simulink model "BLDC_Openloop"  (R2013a)
settings: Solver=ode45  StartTime=0.0  StopTime=0.5  RelTol=1e-3
undefined symbols (not defined in the file or in its folder): DiscIntNeverNeededParam
libraries: simulink x45, powerlib_meascontrol x11, powerlib x9
settings Model: Creator=Sony  LastModifiedBy=Sony

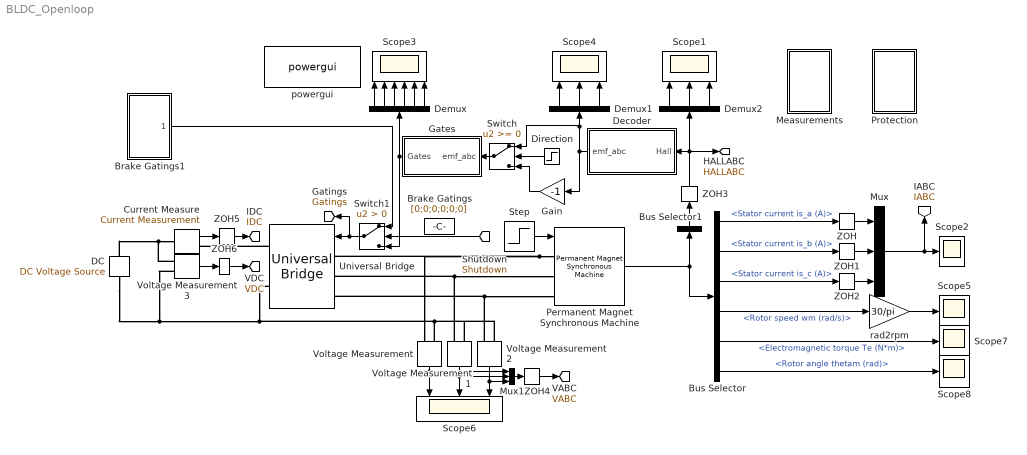
== system BLDC_Openloop ==
  Brake Gatings : Constant  Value=[0;0;0;0;0;0]
  Brake Gatings1 : Subsystem
  Bus Selector : BusSelector  OutputSignals=Stator current is_a (A),Stator current is_b (A),Stator current is_c (A),Rotor speed wm (rad/s),Electromagnetic torque Te (N*m),Rotor angle thetam (rad)
  Bus Selector1 : BusSelector  OutputSignals=Hall effect signal h_a,Hall effect signal h_b,Hall effect signal h_c  OutputAsBus=on
  Current Measure : powerlib/Measurements/Current Measurement  PhasorSimulation=off  OutputType=Complex  PSBequivalent=0
  DC : powerlib/Electrical Sources/DC Voltage Source  Amplitude=48  Measurements=None
  Decoder : Subsystem
  Demux : Demux  Outputs=6
  Demux1 : Demux  Outputs=3
  Demux2 : Demux  Outputs=3
  Direction : Step  Time=.25  Before=1  After=-1  SampleTime=0
  Gain : Gain  Gain=-1
  Gates : Subsystem
  Measurements : Subsystem  mask{Ts=1e-4, Rs=0.01, Ls=1e-4, P=4}
      mask prompts: Ts "Sample Time"; Rs "Stator Resistance"; Ls "Stator Inductance"; P "Pole Pairs"
  Mux : Mux  Inputs=3
  Mux1 : Mux  Inputs=3
  Permanent Magnet Synchronous Machine : powerlib/Machines/Permanent Magnet Synchronous Machine  NbPhases=3  FluxDistribution=Trapezoidal  RotorType=Round  MechanicalLoad=Torque Tm  PresetModel=No  ShowDetailedParameters=on  Resistance=0.01  Inductance=1e-4  dqInductances=[8.5e-3,8.5e-3]  La=0.000835  MachineConstant=Torque Constant (N.m / A_peak)  Flux=0.0125  VoltageCst=10.472  TorqueCst=0.1  Flat=120  Mechanical=[ 1e-3, 1e-7 4]  PolePairs=4  InitialConditions=[(2000)*(pi/30),0, 0,0]  InitialConditions5ph=[0 0 0 0 0 0]  TsPowergui=0  TsBlock=-1  RefAngle=Aligned with phase A axis (original Park)
  Protection : Subsystem  mask{Iphasepeakmax=100, Iphasepeakmin=-100, VDCmax=55, VDCmin=40, IDCmax=125, IDCmin=-125, Accelerationmax=1e7, Accelerationmin=-1e7, VDCrated=48, Temperaturemax=100, Stalltimemax=1, Speedmax=7000, Risetimemax=1e-3}
      mask prompts: Iphasepeakmax "Maximum Phase Peak Current (A)"; Iphasepeakmin "Minimum Phase Peak Current (A)"; VDCmax "Maximum input DC Voltage (V)"; VDCmin "Minimum input DC Voltage (V)"; IDCmax "Maximum input DC Current (A)"; IDCmin "Minimum input DC Current (A)"; Accelerationmax "Maximum Acceleration (rpm/s)"; Accelerationmin "Maximum Deceleration (rpm/s)"; VDCrated "Rated DC input voltage (V)"; Temperaturemax "Maximum Temperature (C)"; Stalltimemax "Maximum Allowed Stall Time (s)"; Speedmax "Maximum Speed (rpm)"; Risetimemax "Maximum MOSFET switch on time (s)"
  Scope1 : Scope  NumInputPorts=3
      settings: YMin=-0.5~-0.5~-0.5  YMax=1.5~1.5~1.5  SaveName=ScopeData3
  Scope{2,5,7..8} (4 alike) : Scope
      Scope2 settings: YMin=-200  YMax=200
      Scope5 settings: YMin=0  YMax=5000  SaveName=ScopeData5
      Scope7 settings: YMin=0  YMax=70  SaveName=ScopeData9
      Scope8 settings: YMin=0  YMax=20  SaveName=ScopeData13
  Scope3 : Scope  NumInputPorts=6
      settings: YMin=-0.5~-0.5~-0.5~-0.5~-0.5~-0.5  YMax=1.5~1.5~1.5~1.5~1.5~1.5
  Scope4 : Scope  NumInputPorts=3
      settings: YMin=-1.5~-1.5~-1.5  YMax=1.5~1.5~1.5  SaveName=ScopeData4
  Scope6 : Scope  NumInputPorts=3
      settings: YMin=-10~-10~-10  YMax=50~50~50  SaveName=ScopeData2
  Step : Step  Time=0.1  After=0  SampleTime=0
  Switch : Switch
  Switch1 : Switch  Criteria=u2 > Threshold
  Universal Bridge : powerlib/Power Electronics/Universal Bridge  Arms=3  SnubberResistance=5000  SnubberCapacitance=1e-6  Device=MOSFET / Diodes  Ron=1e-3  Lon=0  ForwardVoltages="[  0  0  ]"  ForwardVoltage=0  GTOparameters=[ 10e-6 , 20e-6 ]  IGBTparameters=[ 1e-6 , 2e-6 ]  Measurements=None  Measurements_2=None  converterType=Rectifier
  Voltage Measurement{,1..3} (4 alike) : powerlib/Measurements/Voltage Measurement  PhasorSimulation=off  OutputType=Complex  PSBequivalent=0
  ZOH{,1..6} (7 alike) : ZeroOrderHold  SampleTime=1e-4
  powergui : powerlib/powergui  Priority=2  SimulationMode=Discrete  SolverType=Backward Euler  SampleTime=1e-6  frequency=60  SPID=off  DisableSnubberDevices=off  DisableRonSwitches=off  DisableVfSwitches=off  SwTol=0  Interpol=off  DisplayEquations=off  frequencyindice=0  Pbase=100e6  ErrMax=1e-4  Iterations=50  UnitsV=kV  UnitsW=MW  FunctionMessages=off  echomessages=off  HookPort=off  EnableUseOfTLC=off  x0status=blocks  RestoreLinks=warning  ResistiveCurrentMeasurement=off  Frange=[0:2:500]  Ylog=off  Xlog=on  ShowGrid=off  save=off  variable=ZData  ZoomFFT=on  StartTime=0.0  cycles=1  DisplayStyle=1  fundamental=60  FreqAxis=off  MaxFrequency=1000  frequencyindicesteady=1  RmsSteady=1  display=off  Ts=0  methode=off
  rad2rpm : Gain  Gain=30/pi
  tag scope: Gatings=global, HALLABC=global, IABC=global, IDC=global, VABC=global, VDC=global
  wires:
  Step/1 -> Permanent Magnet Synchronous Machine/1
  Gates/1(Gates) -> Switch1/3, Demux/1
  Decoder/1(emf_abc) -> Switch/1, Demux1/1, Gain/1
  rad2rpm/1 -> Scope5/1
  Voltage Measurement/1 -> Mux1/1, Scope6/1
  Bus Selector/1 -> ZOH/1  "<Stator current is_a (A)>"
  Permanent Magnet Synchronous Machine/1 -> Bus Selector/1, Bus Selector1/1
  Bus Selector/2 -> ZOH1/1  "<Stator current is_b (A)>"
  Bus Selector/4 -> rad2rpm/1  "<Rotor speed wm (rad/s)>"
  Demux/3 -> Scope3/3
  Demux/2 -> Scope3/2
  Demux/1 -> Scope3/1
  Demux/4 -> Scope3/4
  Demux/5 -> Scope3/5
  Demux/6 -> Scope3/6
  Demux1/3 -> Scope4/3
  Demux1/2 -> Scope4/2
  Demux1/1 -> Scope4/1
  Demux2/3 -> Scope1/3
  Demux2/2 -> Scope1/2
  Demux2/1 -> Scope1/1
  Bus Selector/3 -> ZOH2/1  "<Stator current is_c (A)>"
  Gain/1 -> Switch/3
  Switch/1 -> Gates/1("emf_abc ")
  Direction/1 -> Switch/2
  Mux/1 -> Scope2/1, [IABC]
  Voltage Measurement1/1 -> Scope6/2, Mux1/2
  Voltage Measurement2/1 -> Scope6/3, Mux1/3
  ZOH/1 -> Mux/1
  ZOH1/1 -> Mux/2
  ZOH2/1 -> Mux/3
  Mux1/1 -> ZOH4/1
  Bus Selector1/1 -> ZOH3/1
  ZOH3/1 -> Demux2/1, [HALLABC], Decoder/1("Hall ")
  Current Measure/1 -> ZOH5/1
  ZOH4/1 -> [VABC]
  Voltage Measurement3/1 -> ZOH6/1
  Bus Selector/5 -> Scope7/1  "<Electromagnetic torque Te (N*m)>"
  ZOH5/1 -> [IDC]
  ZOH6/1 -> [VDC]
  Bus Selector/6 -> Scope8/1  "<Rotor angle thetam (rad)>"
  [Shutdown] -> Switch1/2
  Switch1/1 -> [Gatings], Universal Bridge/1
  Brake Gatings1/1(Gatings) -> Switch1/1
  connections:
  Permanent Magnet Synchronous Machine/LConn1 -- Universal Bridge/LConn1 -- Voltage Measurement/LConn1
  Voltage Measurement1/LConn1 -- Universal Bridge/LConn2 -- Permanent Magnet Synchronous Machine/LConn2
  Voltage Measurement2/LConn1 -- Universal Bridge/LConn3 -- Permanent Magnet Synchronous Machine/LConn3
  DC/RConn1 -- Voltage Measurement3/LConn1 -- Current Measure/LConn1
  DC/LConn1 -- Voltage Measurement3/LConn2 -- Universal Bridge/RConn2 -- Voltage Measurement/LConn2 -- Voltage Measurement1/LConn2 -- Voltage Measurement2/LConn2
  Universal Bridge/RConn1 -- Current Measure/RConn1

== system BLDC_Openloop/Brake Gatings1 ==
  Brake Gatings : Constant  Value=[1;1;1]
  Compare To Zero : simulink/Logic and Bit Operations/Compare To Zero  relop=>=  OutDataTypeStr=boolean
  Constant : Constant  Value=0
  Gates : Subsystem
  Sum2 : Sum  Inputs=|+-
  TRI : powerlib_meascontrol/Pulse & Signal Generators/Triangle Generator  Freq=1e4  Phase=0  Ts=0
  Gatings : Outport
  wires:
  Compare To Zero/1 -> Gates/2(PWM)
  Gates/1(Gates) -> Gatings/1
  Sum2/1 -> Compare To Zero/1
  TRI/1 -> Sum2/2
  Brake Gatings/1 -> Gates/1("emf_abc ")
  Constant/1 -> Sum2/1

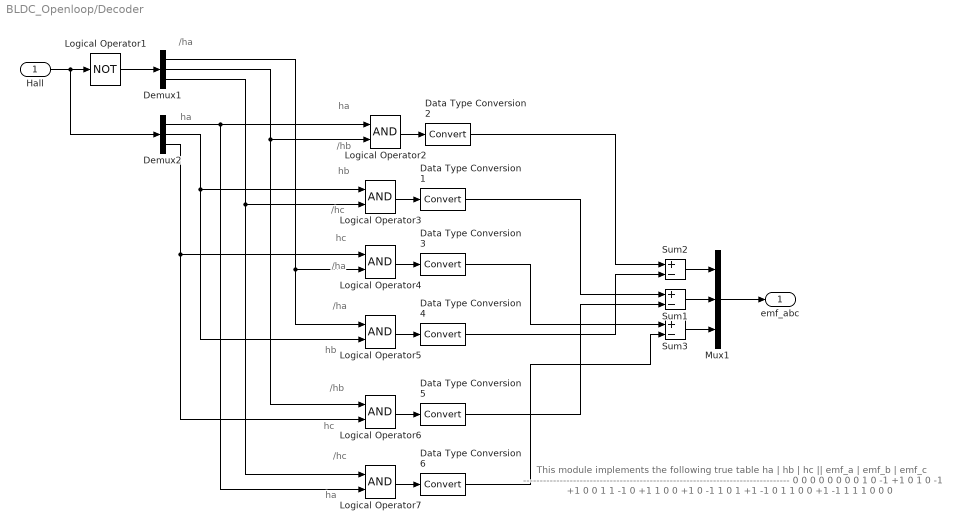
== system BLDC_Openloop/Decoder ==
  note: /ha
  note: ha
  note: ha
  note: /hb
  note: hb
  note: /hc
  note: hc
  note: /ha
  note: /ha
  note: hb
  note: /hb
  note: hc
  note: /hc
  note: ha
  note: This module implements the following true table
      |
      |    ha   |   hb   |   hc   ||   emf_a   |   emf_b   |   emf_c
      |     --------------------------------------------------------------------------------
      | 0          0         0          0               0               0
      | 0          0         1          0               -1              +1
      | 0          1         0          -1              +1                0
      | 0          1         1          -1               0               +1
      | 1          0         0         +1               0               -1
      | 1          0         1         +1              -1                0
      | 1          1         0          0              +1               -1
      | 1          1         1          0               0                0
  "Hall " : Inport
  Data Type Conversion{1..6} (6 alike) : DataTypeConversion
  Demux1 : Demux  Outputs=3
  Demux2 : Demux  Outputs=3
  Logical Operator1 : Logic  Operator=NOT  AllPortsSameDT=off  OutDataTypeStr=boolean
  Logical Operator{2..7} (6 alike) : Logic  AllPortsSameDT=off  OutDataTypeStr=boolean
  Mux1 : Mux  Inputs=3
  Sum1 : Sum  Inputs=+-  OutDataTypeStr=double
  Sum2 : Sum  Inputs=+-  OutDataTypeStr=double
  Sum3 : Sum  Inputs=+-  OutDataTypeStr=double
  emf_abc : Outport
  wires:
  "Hall "/1 -> Logical Operator1/1, Demux2/1
  Logical Operator1/1 -> Demux1/1
  Demux2/3 -> Logical Operator4/1, Logical Operator6/2
  Demux2/2 -> Logical Operator3/1, Logical Operator5/2
  Demux2/1 -> Logical Operator2/1, Logical Operator7/2
  Demux1/3 -> Logical Operator3/2, Logical Operator7/1
  Demux1/2 -> Logical Operator2/2, Logical Operator6/1
  Demux1/1 -> Logical Operator4/2, Logical Operator5/1
  Logical Operator2/1 -> Data Type Conversion2/1
  Sum2/1 -> Mux1/1
  Sum1/1 -> Mux1/2
  Sum3/1 -> Mux1/3
  Mux1/1 -> emf_abc/1
  Logical Operator3/1 -> Data Type Conversion1/1
  Logical Operator4/1 -> Data Type Conversion3/1
  Logical Operator5/1 -> Data Type Conversion4/1
  Logical Operator6/1 -> Data Type Conversion5/1
  Logical Operator7/1 -> Data Type Conversion6/1
  Data Type Conversion2/1 -> Sum2/1
  Data Type Conversion4/1 -> Sum2/2
  Data Type Conversion1/1 -> Sum1/1
  Data Type Conversion5/1 -> Sum1/2
  Data Type Conversion3/1 -> Sum3/1
  Data Type Conversion6/1 -> Sum3/2

== system BLDC_Openloop/Gates ==
  note: This module implements the following true table
      |
      |    emf_a   |   emf_b   |   emf_c   ||   Q1   |   Q2   |   Q3   |   Q4   |   Q5   |   Q6
      |     ------------------------------------------------------------------------------------------------------------------
      |       0              0                0            0          0          0           0        0        0
      |       0               -1              +1          0          0          0           1        1        0
      |     -1              +1                0          0          1          1           0        0        0
      |     -1               0               +1          0          1         0           0        1        0
      |    +1               0                -1          1          0          0           0        0        1
      |    +1              -1                0           1          0          0           1        0        0
      |      0              +1               -1           0          0          1           0        0        1
      |     0              0                0             0          0          0           0        0        0
  "emf_abc " : Inport
  Compare To Zero : simulink/Logic and Bit Operations/Compare To Zero  relop=>  OutDataTypeStr=boolean  ZeroCross=off
  Compare To Zero1 : simulink/Logic and Bit Operations/Compare To Zero  relop=<  OutDataTypeStr=boolean  ZeroCross=off
  Compare To Zero2 : simulink/Logic and Bit Operations/Compare To Zero  relop=>  OutDataTypeStr=boolean  ZeroCross=off
  Compare To Zero3 : simulink/Logic and Bit Operations/Compare To Zero  relop=<  OutDataTypeStr=boolean  ZeroCross=off
  Compare To Zero4 : simulink/Logic and Bit Operations/Compare To Zero  relop=>  OutDataTypeStr=boolean  ZeroCross=off
  Compare To Zero5 : simulink/Logic and Bit Operations/Compare To Zero  relop=<  OutDataTypeStr=boolean  ZeroCross=off
  Demux2 : Demux  Outputs=3
  Mux3 : Mux  Inputs=6
  Gates : Outport
  wires:
  "emf_abc "/1 -> Demux2/1
  Mux3/1 -> Gates/1
  Demux2/1 -> Compare To Zero/1, Compare To Zero1/1
  Demux2/2 -> Compare To Zero2/1, Compare To Zero3/1
  Demux2/3 -> Compare To Zero4/1, Compare To Zero5/1
  Compare To Zero/1 -> Mux3/1
  Compare To Zero1/1 -> Mux3/2
  Compare To Zero2/1 -> Mux3/3
  Compare To Zero3/1 -> Mux3/4
  Compare To Zero4/1 -> Mux3/5
  Compare To Zero5/1 -> Mux3/6

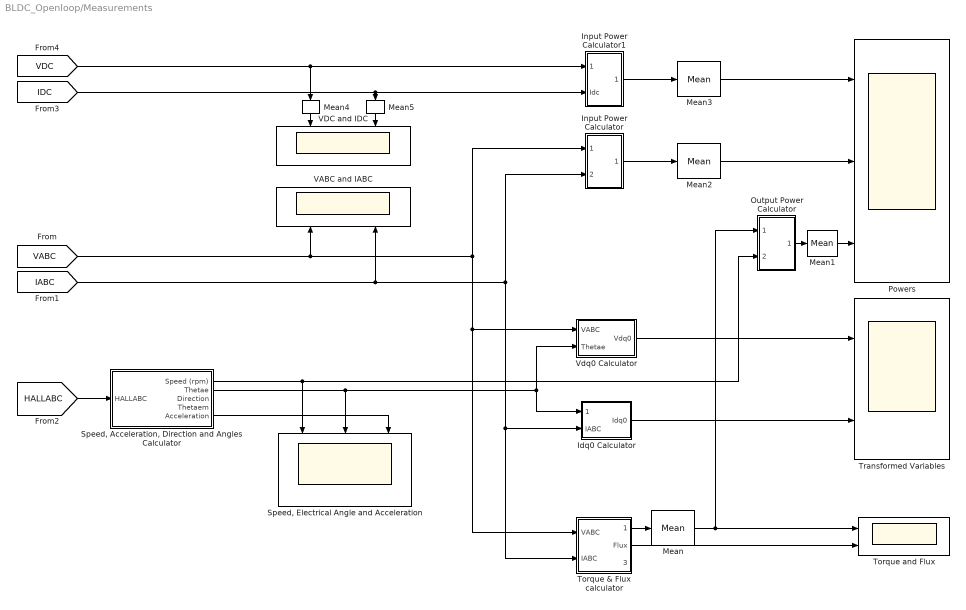
== system BLDC_Openloop/Measurements ==
  Idq0 Calculator : Subsystem
  Input Power Calculator : Subsystem
  Input Power Calculator1 : Subsystem
  Mean{,1..5} (6 alike) : powerlib_meascontrol/Measurements/Mean  Freq=10  Vinit=0  Ts=0
  Output Power Calculator : Subsystem
  Powers : Scope  NumInputPorts=3
      settings: TimeRange=0.5  YMin=0~0~0  YMax=6000~6000~375  SaveName=ScopeData6
  "Speed, Acceleration, Direction and Angles Calculator" : Subsystem
  "Speed, Electrical Angle and Acceleration" : Scope  NumInputPorts=3
      settings: YMin=-10~-7~-2  YMax=8000~7~2  SaveName=ScopeData12
  Torque & Flux calculator : Subsystem  AncestorBlock=electricdrivelib/AC drives/DTC Induction Motor Drive/DTC/Torque & Flux calculator  mask{Rss=Rs, P=P, Ts=Ts}
  Torque and Flux : Scope  NumInputPorts=2
      settings: YMin=0~0  YMax=20~0.1  SaveName=ScopeData10
  Transformed Variables : Scope  NumInputPorts=2
      settings: YMin=-35~-800  YMax=35~800  SaveName=ScopeData7
  VABC and IABC : Scope  NumInputPorts=2
      settings: YMin=-5~-200  YMax=50~200  SaveName=ScopeData14
  VDC and IDC : Scope  NumInputPorts=2
      settings: YMin=45.6~0  YMax=50.4~100  SaveName=ScopeData15
  Vdq0 Calculator : Subsystem
  wires:
  [HALLABC] -> "Speed, Acceleration, Direction and Angles Calculator"/1(HALLABC)
  "Speed, Acceleration, Direction and Angles Calculator"/2(Thetae) -> "Speed, Electrical Angle and Acceleration"/2, Idq0 Calculator/1(Thetae), Vdq0 Calculator/2(Thetae)
  [VABC] -> VABC and IABC/1, Input Power Calculator/1(Vabc), Torque & Flux calculator/1(VABC), Vdq0 Calculator/1(VABC)
  [IABC] -> VABC and IABC/2, Input Power Calculator/2(Iabc), Torque & Flux calculator/2(IABC), Idq0 Calculator/2(IABC)
  Torque & Flux calculator/1(Torque) -> Mean/1
  Input Power Calculator/1(Pin) -> Mean2/1
  [VDC] -> Input Power Calculator1/1(Vdc), Mean4/1
  [IDC] -> Input Power Calculator1/2(Idc), Mean5/1
  Input Power Calculator1/1(Pin) -> Mean3/1
  Output Power Calculator/1(Pout) -> Mean1/1
  Vdq0 Calculator/1(Vdq0) -> Transformed Variables/1
  Idq0 Calculator/1(Idq0) -> Transformed Variables/2
  Torque & Flux calculator/2(Flux) -> Torque and Flux/2
  "Speed, Acceleration, Direction and Angles Calculator"/1(Speed (rpm)) -> Output Power Calculator/2(Speed), "Speed, Electrical Angle and Acceleration"/1
  "Speed, Acceleration, Direction and Angles Calculator"/5(Acceleration) -> "Speed, Electrical Angle and Acceleration"/3
  Mean/1 -> Output Power Calculator/1(Torque), Torque and Flux/1
  Mean1/1 -> Powers/3
  Mean2/1 -> Powers/2
  Mean3/1 -> Powers/1
  Mean4/1 -> VDC and IDC/1
  Mean5/1 -> VDC and IDC/2

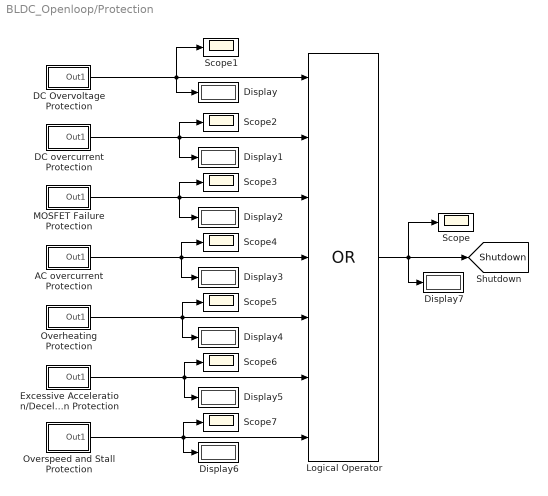
== system BLDC_Openloop/Protection ==
  AC overcurrent Protection : Subsystem
  DC Overvoltage Protection : Subsystem
  DC overcurrent Protection : Subsystem
  Display{,1..7} (8 alike) : Display
  Excessive Acceleration/Deceleration Protection : Subsystem
  Logical Operator : Logic  Operator=OR  Inputs=7  AllPortsSameDT=off  OutDataTypeStr=boolean
  MOSFET Failure Protection : Subsystem
  Overheating Protection : Subsystem
  Overspeed and Stall Protection : Subsystem
  Scope{,1..7} (8 alike) : Scope
      Scope settings: SaveName=ScopeData18
      Scope1 settings: SaveName=ScopeData19
      Scope2 settings: SaveName=ScopeData20
      Scope3 settings: SaveName=ScopeData21
      Scope4 settings: SaveName=ScopeData22
      Scope5 settings: SaveName=ScopeData23
      Scope6 settings: SaveName=ScopeData24
      Scope7 settings: SaveName=ScopeData25
  tag scope: Shutdown=global
  wires:
  DC Overvoltage Protection/1(Out1) -> Scope1/1, Display/1, Logical Operator/1
  DC overcurrent Protection/1(Out1) -> Scope2/1, Display1/1, Logical Operator/2
  MOSFET Failure Protection/1(Out1) -> Logical Operator/3, Scope3/1, Display2/1
  AC overcurrent Protection/1(Out1) -> Scope4/1, Display3/1, Logical Operator/4
  Overheating Protection/1(Out1) -> Display4/1, Scope5/1, Logical Operator/5
  Excessive Acceleration/Deceleration Protection/1(Out1) -> Scope6/1, Display5/1, Logical Operator/6
  Overspeed and Stall Protection/1(Out1) -> Scope7/1, Logical Operator/7, Display6/1
  Logical Operator/1 -> Scope/1, Display7/1, [Shutdown]

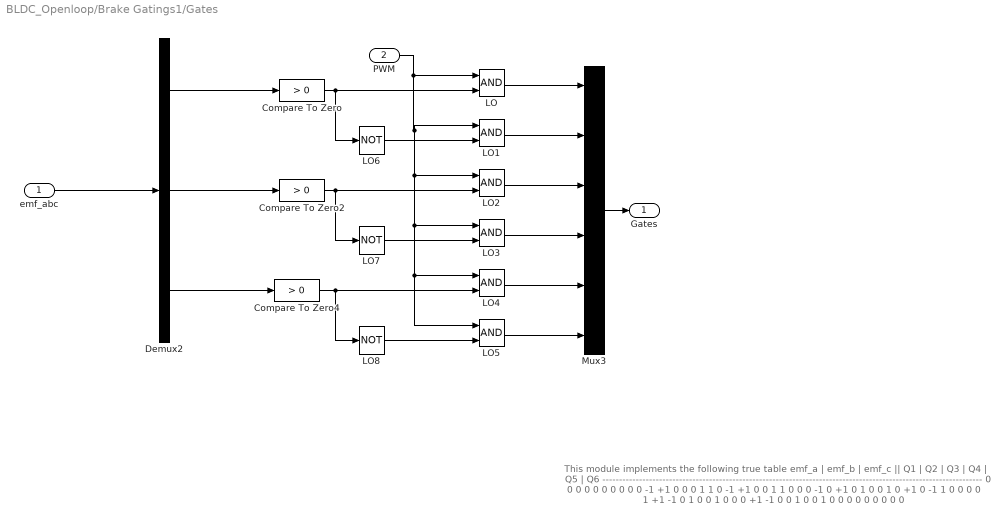
== system BLDC_Openloop/Brake Gatings1/Gates ==
  note: This module implements the following true table
      |
      |    emf_a   |   emf_b   |   emf_c   ||   Q1   |   Q2   |   Q3   |   Q4   |   Q5   |   Q6
      |     ------------------------------------------------------------------------------------------------------------------
      |       0              0                0            0          0          0           0        0        0
      |       0               -1              +1          0          0          0           1        1        0
      |     -1              +1                0          0          1          1           0        0        0
      |     -1               0               +1          0          1         0           0        1        0
      |    +1               0                -1          1          0          0           0        0        1
      |    +1              -1                0           1          0          0           1        0        0
      |      0              +1               -1           0          0          1           0        0        1
      |     0              0                0             0          0          0           0        0        0
  "emf_abc " : Inport
  PWM : Inport  Port=2
  Compare To Zero : simulink/Logic and Bit Operations/Compare To Zero  relop=>  OutDataTypeStr=boolean  ZeroCross=off
  Compare To Zero2 : simulink/Logic and Bit Operations/Compare To Zero  relop=>  OutDataTypeStr=boolean  ZeroCross=off
  Compare To Zero4 : simulink/Logic and Bit Operations/Compare To Zero  relop=>  OutDataTypeStr=boolean  ZeroCross=off
  Demux2 : Demux  Outputs=3
  LO{,1..5} (6 alike) : Logic  AllPortsSameDT=off  OutDataTypeStr=boolean
  LO6 : Logic  Operator=NOT  AllPortsSameDT=off  OutDataTypeStr=boolean
  LO7 : Logic  Operator=NOT  AllPortsSameDT=off  OutDataTypeStr=boolean
  LO8 : Logic  Operator=NOT  AllPortsSameDT=off  OutDataTypeStr=boolean
  Mux3 : Mux  Inputs=6
  Gates : Outport
  wires:
  "emf_abc "/1 -> Demux2/1
  Mux3/1 -> Gates/1
  Demux2/1 -> Compare To Zero/1
  Demux2/2 -> Compare To Zero2/1
  Demux2/3 -> Compare To Zero4/1
  LO/1 -> Mux3/1
  LO6/1 -> LO1/2
  Compare To Zero/1 -> LO6/1, LO/2
  PWM/1 -> LO/1, LO5/1, LO4/1, LO3/1, LO2/1, LO1/1
  LO1/1 -> Mux3/2
  Compare To Zero2/1 -> LO7/1, LO2/2
  LO2/1 -> Mux3/3
  LO7/1 -> LO3/2
  Compare To Zero4/1 -> LO8/1, LO4/2
  LO8/1 -> LO5/2
  LO5/1 -> Mux3/6
  LO4/1 -> Mux3/5
  LO3/1 -> Mux3/4

== system BLDC_Openloop/Measurements/Idq0 Calculator ==
  Thetae : Inport
  IABC : Inport  Port=2
  abc to dq0 : powerlib_meascontrol/Transformations/abc to dq0  Alignment=Aligned with phase A axis
  Idq0 : Outport
  wires:
  IABC/1 -> abc to dq0/1
  Thetae/1 -> abc to dq0/2
  abc to dq0/1 -> Idq0/1

== system BLDC_Openloop/Measurements/Input Power Calculator ==
  Vabc : Inport
  Iabc : Inport  Port=2
  Product : Product
  Sum of Elements : Sum  Inputs=+
  Pin : Outport
  wires:
  Vabc/1 -> Product/1
  Product/1 -> Sum of Elements/1
  Iabc/1 -> Product/2
  Sum of Elements/1 -> Pin/1

== system BLDC_Openloop/Measurements/Input Power Calculator1 ==
  Vdc : Inport
  Idc : Inport  Port=2
  Product : Product
  Pin : Outport
  wires:
  Vdc/1 -> Product/1
  Product/1 -> Pin/1
  Idc/1 -> Product/2

== system BLDC_Openloop/Measurements/Output Power Calculator ==
  Torque : Inport
  Speed : Inport  Port=2
  Gain : Gain  Gain=pi/30
  Product : Product
  Pout : Outport
  wires:
  Torque/1 -> Product/1
  Product/1 -> Pout/1
  Speed/1 -> Gain/1
  Gain/1 -> Product/2

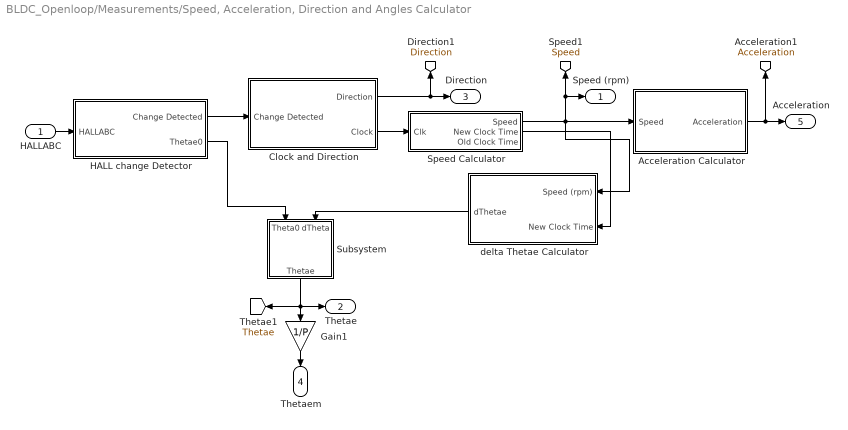
== system BLDC_Openloop/Measurements/Speed, Acceleration, Direction and Angles Calculator ==
  HALLABC : Inport
  Acceleration Calculator : Subsystem
  Clock and Direction : Subsystem
  Gain1 : Gain  Gain=1/P
  HALL change Detector : Subsystem
  Speed Calculator : Subsystem
  Subsystem : Subsystem
  delta Thetae Calculator : Subsystem
  Speed (rpm) : Outport
  Thetae : Outport  Port=2
  Direction : Outport  Port=3
  Thetaem : Outport  Port=4
  Acceleration : Outport  Port=5
  tag scope: Acceleration=global, Direction=global, Speed=global, Thetae=global
  wires:
  HALLABC/1 -> HALL change Detector/1(HALLABC)
  Clock and Direction/2(Clock) -> Speed Calculator/1(Clk)
  HALL change Detector/1(Change Detected) -> Clock and Direction/1(Change Detected)
  Clock and Direction/1(Direction) -> Direction/1, [Direction]
  Speed Calculator/2(New Clock Time) -> delta Thetae Calculator/2(New Clock Time)
  Acceleration Calculator/1(Acceleration) -> [Acceleration], Acceleration/1
  Speed Calculator/1(Speed) -> delta Thetae Calculator/1(Speed (rpm)), Acceleration Calculator/1(Speed), Speed (rpm)/1, [Speed]
  HALL change Detector/2(Thetae0) -> Subsystem/1(Theta0)
  delta Thetae Calculator/1(dThetae) -> Subsystem/2(dTheta)
  Gain1/1 -> Thetaem/1
  Subsystem/1(Thetae) -> Thetae/1, Gain1/1, [Thetae]

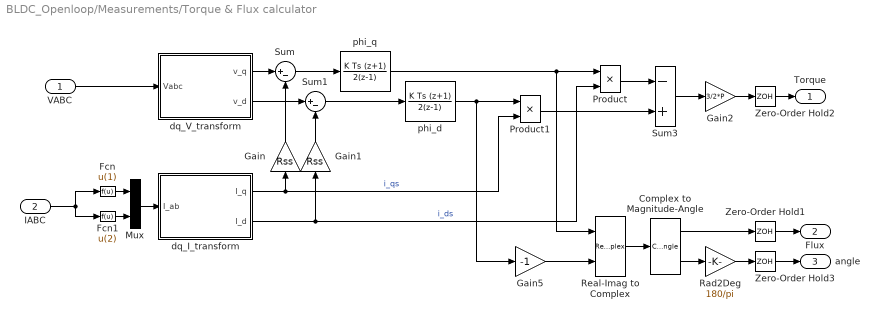
== system BLDC_Openloop/Measurements/Torque & Flux calculator ==
  VABC : Inport
  IABC : Inport  Port=2
  Complex to Magnitude-Angle : ComplexToMagnitudeAngle
  Fcn : Fcn  Expr=u(1)
  Fcn1 : Fcn  Expr=u(2)
  Gain : Gain  Gain=Rss  SaturateOnIntegerOverflow=on  OutDataTypeStr=Inherit: Same as input  ParamDataTypeStr=Inherit: Same as input
  Gain1 : Gain  Gain=Rss  SaturateOnIntegerOverflow=on  OutDataTypeStr=Inherit: Same as input  ParamDataTypeStr=Inherit: Same as input
  Gain2 : Gain  Gain=3/2*P  SaturateOnIntegerOverflow=on  OutDataTypeStr=Inherit: Same as input  ParamDataTypeStr=Inherit: Same as input
  Gain5 : Gain  Gain=-1  SaturateOnIntegerOverflow=on  OutDataTypeStr=Inherit: Same as input  ParamDataTypeStr=Inherit: Same as input
  Mux : Mux  Inputs=2
  Product : Product  SaturateOnIntegerOverflow=on  OutDataTypeStr=Inherit: Same as first input
  Product1 : Product  SaturateOnIntegerOverflow=on  OutDataTypeStr=Inherit: Same as first input
  Rad2Deg : Gain  Gain=180/pi  SaturateOnIntegerOverflow=on  OutDataTypeStr=Inherit: Same as input  ParamDataTypeStr=Inherit: Same as input
  Real-Imag to Complex : RealImagToComplex
  Sum : Sum  Inputs=|+-  SaturateOnIntegerOverflow=on
  Sum1 : Sum  Inputs=|+-  SaturateOnIntegerOverflow=on
  Sum3 : Sum  Inputs=-+  SaturateOnIntegerOverflow=on
  Zero-Order Hold1 : ZeroOrderHold  SampleTime=Ts
  Zero-Order Hold2 : ZeroOrderHold  SampleTime=Ts
  Zero-Order Hold3 : ZeroOrderHold  SampleTime=Ts
  dq_I_transform : Subsystem
  dq_V_transform : Subsystem
  phi_d : DiscreteIntegrator  IntegratorMethod=Integration: Trapezoidal  SampleTime=Ts  ICPrevOutput=DiscIntNeverNeededParam  ICPrevScaledInput=DiscIntNeverNeededParam
  phi_q : DiscreteIntegrator  IntegratorMethod=Integration: Trapezoidal  SampleTime=Ts  ICPrevOutput=DiscIntNeverNeededParam  ICPrevScaledInput=DiscIntNeverNeededParam
  Torque : Outport
  Flux : Outport  Port=2
  angle : Outport  Port=3
  wires:
  Zero-Order Hold3/1 -> angle/1
  Zero-Order Hold1/1 -> Flux/1
  Zero-Order Hold2/1 -> Torque/1
  Product1/1 -> Sum3/2
  Gain5/1 -> Real-Imag to Complex/2
  Rad2Deg/1 -> Zero-Order Hold3/1
  Complex to Magnitude-Angle/2 -> Rad2Deg/1
  Complex to Magnitude-Angle/1 -> Zero-Order Hold1/1
  Real-Imag to Complex/1 -> Complex to Magnitude-Angle/1
  VABC/1 -> dq_V_transform/1(Vabc)
  dq_V_transform/1(v_q) -> Sum/1
  dq_I_transform/1(I_q) -> Gain/1, Product1/2  "i_qs"
  Gain/1 -> Sum/2
  Sum/1 -> phi_q/1
  dq_V_transform/2(v_d) -> Sum1/1
  Gain1/1 -> Sum1/2
  dq_I_transform/2(I_d) -> Product/2, Gain1/1  "i_ds"
  Sum1/1 -> phi_d/1
  phi_q/1 -> Real-Imag to Complex/1, Product/1
  phi_d/1 -> Gain5/1, Product1/1
  Product/1 -> Sum3/1
  Sum3/1 -> Gain2/1
  Gain2/1 -> Zero-Order Hold2/1
  IABC/1 -> Fcn1/1, Fcn/1
  Mux/1 -> dq_I_transform/1(I_ab)
  Fcn/1 -> Mux/1
  Fcn1/1 -> Mux/2

== system BLDC_Openloop/Measurements/Vdq0 Calculator ==
  VABC : Inport
  Thetae : Inport  Port=2
  abc to dq1 : powerlib_meascontrol/Transformations/abc to dq0  Alignment=Aligned with phase A axis
  Vdq0 : Outport
  wires:
  abc to dq1/1 -> Vdq0/1
  Thetae/1 -> abc to dq1/2
  VABC/1 -> abc to dq1/1

== system BLDC_Openloop/Protection/AC overcurrent Protection ==
  C5 : simulink/Logic and Bit Operations/Compare To Constant  relop=>=  const=Iphasepeakmax  OutDataTypeStr=boolean
  C7 : simulink/Logic and Bit Operations/Compare To Constant  relop=>=  const=Iphasepeakmax  OutDataTypeStr=boolean
  C8 : simulink/Logic and Bit Operations/Compare To Constant  relop=>=  const=Iphasepeakmax  OutDataTypeStr=boolean
  Demux : Demux  Outputs=3
  Logical Operator : Logic  Operator=OR  Inputs=3  AllPortsSameDT=off  OutDataTypeStr=boolean
  Out1 : Outport
  wires:
  C5/1 -> Logical Operator/1
  C8/1 -> Logical Operator/3
  C7/1 -> Logical Operator/2
  [IABC] -> Demux/1
  Demux/2 -> C7/1
  Demux/3 -> C8/1
  Demux/1 -> C5/1
  Logical Operator/1 -> Out1/1

== system BLDC_Openloop/Protection/DC Overvoltage Protection ==
  C1 : simulink/Logic and Bit Operations/Compare To Constant  relop=<=  const=VDCmin  OutDataTypeStr=boolean
  C2 : simulink/Logic and Bit Operations/Compare To Constant  relop=>=  const=VDCmax  OutDataTypeStr=boolean
  Logical Operator7 : Logic  Operator=OR  AllPortsSameDT=off  OutDataTypeStr=boolean
  Out1 : Outport
  wires:
  [VDC] -> C2/1, C1/1
  Logical Operator7/1 -> Out1/1
  C1/1 -> Logical Operator7/1
  C2/1 -> Logical Operator7/2

== system BLDC_Openloop/Protection/DC overcurrent Protection ==
  C10 : simulink/Logic and Bit Operations/Compare To Constant  relop=<=  const=IDCmin  OutDataTypeStr=boolean
  C3 : simulink/Logic and Bit Operations/Compare To Constant  relop=>=  const=IDCmax  OutDataTypeStr=boolean
  Logical Operator6 : Logic  Operator=OR  AllPortsSameDT=off  OutDataTypeStr=boolean
  Out1 : Outport
  wires:
  C10/1 -> Logical Operator6/1
  C3/1 -> Logical Operator6/2
  [IDC] -> C10/1, C3/1
  Logical Operator6/1 -> Out1/1

== system BLDC_Openloop/Protection/Excessive Acceleration//Deceleration Protection ==
  C6 : simulink/Logic and Bit Operations/Compare To Constant  relop=<=  const=Accelerationmin  OutDataTypeStr=boolean
  C9 : simulink/Logic and Bit Operations/Compare To Constant  relop=>=  const=Accelerationmax  OutDataTypeStr=boolean
  Logical Operator5 : Logic  Operator=OR  AllPortsSameDT=off  OutDataTypeStr=boolean
  Scope1 : Scope
      settings: SaveName=ScopeData26
  Scope2 : Scope
      settings: SaveName=ScopeData27
  Scope3 : Scope
      settings: YMin=-1  YMax=1  SaveName=ScopeData28
  Out1 : Outport
  wires:
  C9/1 -> Scope2/1, Logical Operator5/2
  [Acceleration] -> C9/1, Scope3/1, C6/1
  Logical Operator5/1 -> Out1/1
  C6/1 -> Scope1/1, Logical Operator5/1

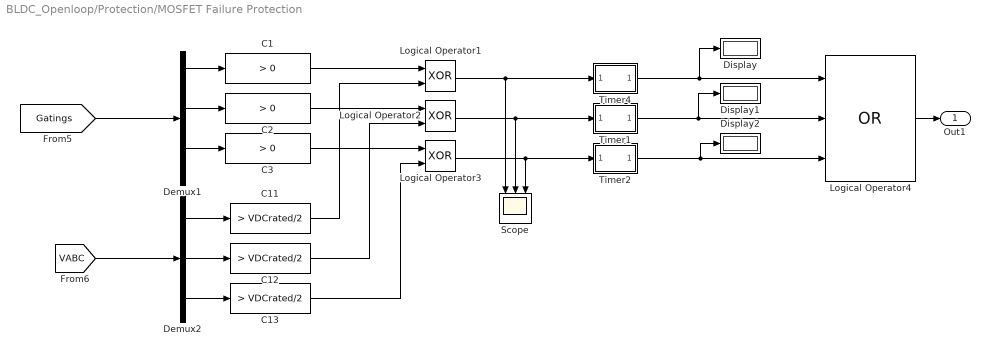
== system BLDC_Openloop/Protection/MOSFET Failure Protection ==
  C1 : simulink/Logic and Bit Operations/Compare To Constant  relop=>  const=0  OutDataTypeStr=boolean
  C11 : simulink/Logic and Bit Operations/Compare To Constant  relop=>  const=VDCrated/2  OutDataTypeStr=boolean
  C12 : simulink/Logic and Bit Operations/Compare To Constant  relop=>  const=VDCrated/2  OutDataTypeStr=boolean
  C13 : simulink/Logic and Bit Operations/Compare To Constant  relop=>  const=VDCrated/2  OutDataTypeStr=boolean
  C2 : simulink/Logic and Bit Operations/Compare To Constant  relop=>  const=0  OutDataTypeStr=boolean
  C3 : simulink/Logic and Bit Operations/Compare To Constant  relop=>  const=0  OutDataTypeStr=boolean
  Demux1 : Demux  Outputs=6
  Demux2 : Demux  Outputs=3
  Display : Display
  Display1 : Display
  Display2 : Display
  Logical Operator1 : Logic  Operator=XOR  AllPortsSameDT=off  OutDataTypeStr=boolean
  Logical Operator2 : Logic  Operator=XOR  AllPortsSameDT=off  OutDataTypeStr=boolean
  Logical Operator3 : Logic  Operator=XOR  AllPortsSameDT=off  OutDataTypeStr=boolean
  Logical Operator4 : Logic  Operator=OR  Inputs=3  AllPortsSameDT=off  OutDataTypeStr=boolean
  Scope : Scope  NumInputPorts=3
      settings: YMin=-5~-5~-5  YMax=5~5~5  SaveName=ScopeData17
  Timer1 : Subsystem
  Timer2 : Subsystem
  Timer4 : Subsystem
  Out1 : Outport
  wires:
  Logical Operator3/1 -> Timer2/1(In1), Scope/3
  Demux2/3 -> C13/1
  Logical Operator2/1 -> Timer1/1(In1), Scope/2
  Demux1/3 -> C2/1
  Demux1/1 -> C1/1
  Demux1/5 -> C3/1
  Demux2/1 -> C11/1
  C13/1 -> Logical Operator3/2
  C11/1 -> Logical Operator1/2
  Demux2/2 -> C12/1
  Logical Operator1/1 -> Timer4/1(In1), Scope/1
  C12/1 -> Logical Operator2/2
  Logical Operator4/1 -> Out1/1
  C1/1 -> Logical Operator1/1
  C2/1 -> Logical Operator2/1
  C3/1 -> Logical Operator3/1
  Timer4/1(Out1) -> Display/1, Logical Operator4/1
  Timer1/1(Out1) -> Display1/1, Logical Operator4/2
  Timer2/1(Out1) -> Display2/1, Logical Operator4/3
  [Gatings] -> Demux1/1
  [VABC] -> Demux2/1

== system BLDC_Openloop/Protection/Overheating Protection ==
  C19 : simulink/Logic and Bit Operations/Compare To Constant  relop=>=  const=Temperaturemax  OutDataTypeStr=boolean
  Out1 : Outport
  wires:
  [Temperature] -> C19/1
  C19/1 -> Out1/1

== system BLDC_Openloop/Protection/Overspeed and Stall Protection ==
  Add2 : Sum  Inputs=+-
  C17 : simulink/Logic and Bit Operations/Compare To Constant  relop===  const=0  OutDataTypeStr=boolean
  C18 : simulink/Logic and Bit Operations/Compare To Constant  relop=>=  const=Stalltimemax  OutDataTypeStr=boolean
  C4 : simulink/Logic and Bit Operations/Compare To Constant  relop=>=  const=Speedmax  OutDataTypeStr=boolean
  Clock : Clock
      settings: Decimation=1000000
  Edge Detector : powerlib_meascontrol/Logic/Edge Detector  model=Rising  ic=0  Ts=0
  Logical Operator8 : Logic  Operator=OR  AllPortsSameDT=off  OutDataTypeStr=boolean
  Scope1 : Scope
      settings: SaveName=ScopeData29
  Scope2 : Scope
      settings: SaveName=ScopeData30
  Switch : Switch  Criteria=u2 > Threshold
  Out1 : Outport
  wires:
  C18/1 -> Scope1/1, Logical Operator8/1
  Logical Operator8/1 -> Out1/1
  [Speed] -> C4/1, C17/1
  Add2/1 -> C18/1
  C17/1 -> Edge Detector/1
  Switch/1 -> Switch/3, Add2/2
  Edge Detector/1 -> Switch/2
  Clock/1 -> Add2/1, Switch/1
  C4/1 -> Scope2/1, Logical Operator8/2

== system BLDC_Openloop/Measurements/Speed, Acceleration, Direction and Angles Calculator/Acceleration Calculator ==
  Speed : Inport
  Add : Sum  Inputs=+-
  Constant : Constant  Value=Ts
  Divide : Product  Inputs=*/
  Zero-Order Hold : ZeroOrderHold  SampleTime=Ts
  Acceleration : Outport
  wires:
  Speed/1 -> Add/1, Zero-Order Hold/1
  Zero-Order Hold/1 -> Add/2
  Add/1 -> Divide/1
  Constant/1 -> Divide/2
  Divide/1 -> Acceleration/1

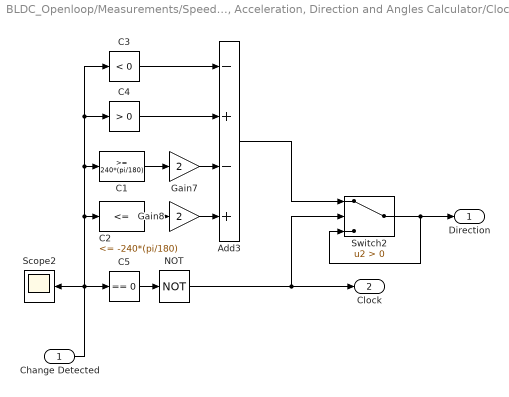
== system BLDC_Openloop/Measurements/Speed, Acceleration, Direction and Angles Calculator/Clock and Direction ==
  Change Detected : Inport
  Add3 : Sum  Inputs=-+-+  OutDataTypeStr=double
  C1 : simulink/Logic and Bit Operations/Compare To Constant  relop=>=  const=240*(pi/180)  OutDataTypeStr=boolean
  C2 : simulink/Logic and Bit Operations/Compare To Constant  relop=<=  const=-240*(pi/180)  OutDataTypeStr=boolean
  C3 : simulink/Logic and Bit Operations/Compare To Zero  relop=<  OutDataTypeStr=boolean
  C4 : simulink/Logic and Bit Operations/Compare To Zero  relop=>  OutDataTypeStr=boolean
  C5 : simulink/Logic and Bit Operations/Compare To Zero  relop===  OutDataTypeStr=boolean
  Gain7 : Gain  Gain=2
  Gain8 : Gain  Gain=2
  NOT : Logic  Operator=NOT  AllPortsSameDT=off  OutDataTypeStr=boolean
  Scope2 : Scope
      settings: YMin=-7  YMax=7  SaveName=ScopeData11
  Switch2 : Switch  Criteria=u2 > Threshold
  Direction : Outport
  Clock : Outport  Port=2
  wires:
  Change Detected/1 -> Scope2/1, C5/1, C2/1, C1/1, C4/1, C3/1
  C3/1 -> Add3/1
  C5/1 -> NOT/1
  Add3/1 -> Switch2/1
  Gain7/1 -> Add3/3
  Gain8/1 -> Add3/4
  NOT/1 -> Switch2/2, Clock/1
  C4/1 -> Add3/2
  C1/1 -> Gain7/1
  C2/1 -> Gain8/1
  Switch2/1 -> Switch2/3, Direction/1

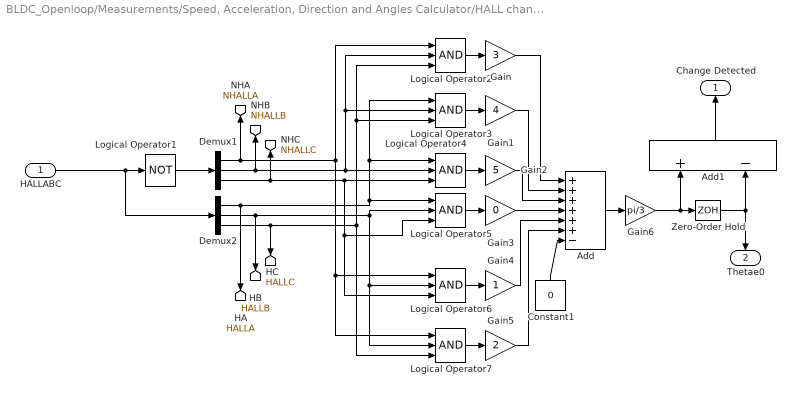
== system BLDC_Openloop/Measurements/Speed, Acceleration, Direction and Angles Calculator/HALL change Detector ==
  HALLABC : Inport
  Add : Sum  Inputs=++++++-
  Add1 : Sum  Inputs=+-
  Constant1 : Constant  Value=0
  Demux1 : Demux  Outputs=3
  Demux2 : Demux  Outputs=3
  Gain : Gain  Gain=3
  Gain1 : Gain  Gain=4
  Gain2 : Gain  Gain=5
  Gain3 : Gain  Gain=0
  Gain4 : Gain
  Gain5 : Gain  Gain=2
  Gain6 : Gain  Gain=pi/3  ParamDataTypeStr=double
  Logical Operator1 : Logic  Operator=NOT  AllPortsSameDT=off  OutDataTypeStr=boolean
  Logical Operator{2..7} (6 alike) : Logic  Inputs=3  AllPortsSameDT=off  OutDataTypeStr=boolean
  Zero-Order Hold : ZeroOrderHold  SampleTime=1.01*Ts
  Change Detected : Outport
  Thetae0 : Outport  Port=2
  tag scope: HALLA=global, HALLB=global, HALLC=global, NHALLA=global, NHALLB=global, NHALLC=global
  wires:
  Logical Operator6/1 -> Gain4/1
  Gain/1 -> Add/1
  Logical Operator3/1 -> Gain1/1
  Gain1/1 -> Add/2
  Add1/1 -> Change Detected/1
  Add/1 -> Gain6/1
  Demux1/1 -> [NHALLA], Logical Operator7/1, Logical Operator6/1, Logical Operator2/1
  Gain2/1 -> Add/3
  Demux2/3 -> Logical Operator7/3, Logical Operator3/3, Logical Operator2/3, [HALLC]
  Demux2/1 -> [HALLA], Logical Operator4/1, Logical Operator3/1, Logical Operator5/1
  Logical Operator1/1 -> Demux1/1
  Logical Operator5/1 -> Gain3/1
  Demux1/2 -> Logical Operator3/2, Logical Operator2/2, Logical Operator4/2, [NHALLB]
  Demux2/2 -> Logical Operator6/2, Logical Operator7/2, Logical Operator5/2, [HALLB]
  Gain4/1 -> Add/5
  Logical Operator4/1 -> Gain2/1
  HALLABC/1 -> Logical Operator1/1, Demux2/1
  Gain6/1 -> Add1/1, Zero-Order Hold/1
  Gain5/1 -> Add/6
  Logical Operator7/1 -> Gain5/1
  Logical Operator2/1 -> Gain/1
  Gain3/1 -> Add/4
  Demux1/3 -> Logical Operator6/3, Logical Operator5/3, Logical Operator4/3, [NHALLC]
  Zero-Order Hold/1 -> Thetae0/1, Add1/2
  Constant1/1 -> Add/7

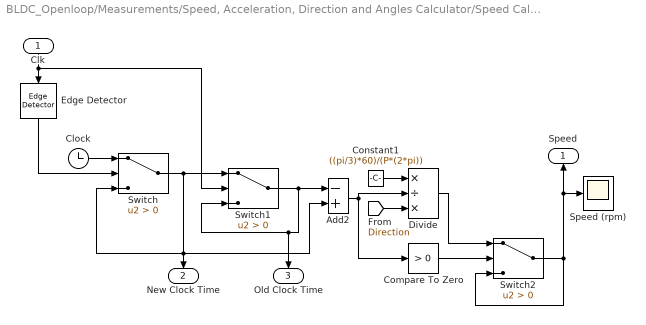
== system BLDC_Openloop/Measurements/Speed, Acceleration, Direction and Angles Calculator/Speed Calculator ==
  Clk : Inport
  Add2 : Sum  Inputs=-+
  Clock : Clock
      settings: Decimation=1000000
  Compare To Zero : simulink/Logic and Bit Operations/Compare To Zero  relop=>  OutDataTypeStr=boolean
  Constant1 : Constant  Value=((pi/3)*60)/(P*(2*pi))
  Divide : Product  Inputs=*/*  LockScale=on
  Edge Detector : powerlib_meascontrol/Logic/Edge Detector  model=Falling  ic=0  Ts=-1
  Speed (rpm) : Scope
      settings: YMin=-5000  YMax=5000  SaveName=ScopeData8
  Switch : Switch  Criteria=u2 > Threshold
  Switch1 : Switch  Criteria=u2 > Threshold
  Switch2 : Switch  Criteria=u2 > Threshold
  Speed : Outport
  New Clock Time : Outport  Port=2
  Old Clock Time : Outport  Port=3
  wires:
  Clk/1 -> Edge Detector/1, Switch1/2
  Divide/1 -> Switch2/1
  Constant1/1 -> Divide/1
  Clock/1 -> Switch/1
  Switch1/1 -> Old Clock Time/1, Switch1/3, Add2/1
  [Direction] -> Divide/3
  Add2/1 -> Compare To Zero/1, Divide/2
  Edge Detector/1 -> Switch/2
  Switch/1 -> Add2/2, New Clock Time/1, Switch/3, Switch1/1
  Compare To Zero/1 -> Switch2/2
  Switch2/1 -> Speed (rpm)/1, Speed/1, Switch2/3

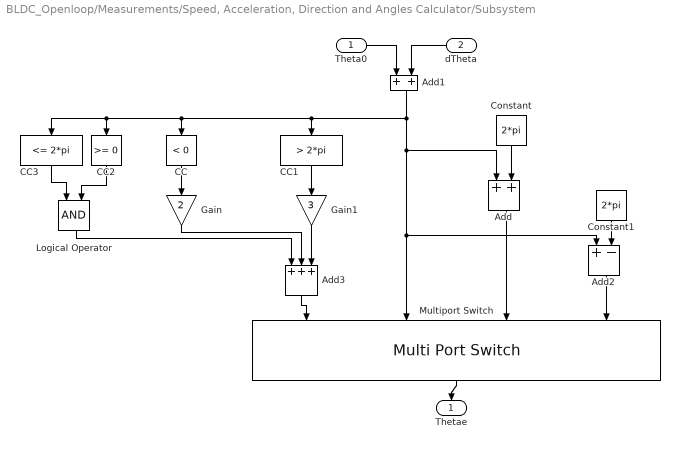
== system BLDC_Openloop/Measurements/Speed, Acceleration, Direction and Angles Calculator/Subsystem ==
  Theta0 : Inport
  dTheta : Inport  Port=2
  Add : Sum
  Add1 : Sum
  Add2 : Sum  Inputs=+-
  Add3 : Sum  Inputs=+++
  CC : simulink/Logic and Bit Operations/Compare To Constant  relop=<  const=0  OutDataTypeStr=boolean
  CC1 : simulink/Logic and Bit Operations/Compare To Constant  relop=>  const=2*pi  OutDataTypeStr=boolean
  CC2 : simulink/Logic and Bit Operations/Compare To Constant  relop=>=  const=0  OutDataTypeStr=boolean
  CC3 : simulink/Logic and Bit Operations/Compare To Constant  relop=<=  const=2*pi  OutDataTypeStr=boolean
  Constant : Constant  Value=2*pi
  Constant1 : Constant  Value=2*pi
  Gain : Gain  Gain=2
  Gain1 : Gain  Gain=3
  Logical Operator : Logic  AllPortsSameDT=off  OutDataTypeStr=boolean
  Multiport Switch : MultiPortSwitch
  Thetae : Outport
  wires:
  Theta0/1 -> Add1/1
  dTheta/1 -> Add1/2
  Constant1/1 -> Add2/2
  Constant/1 -> Add/2
  Add2/1 -> Multiport Switch/4
  Multiport Switch/1 -> Thetae/1
  Add/1 -> Multiport Switch/3
  CC/1 -> Gain/1
  CC1/1 -> Gain1/1
  CC3/1 -> Logical Operator/1
  CC2/1 -> Logical Operator/2
  Add3/1 -> Multiport Switch/1
  Gain1/1 -> Add3/3
  Gain/1 -> Add3/2
  Logical Operator/1 -> Add3/1
  Add1/1 -> CC2/1, CC3/1, CC/1, CC1/1, Add2/1, Multiport Switch/2, Add/1

== system BLDC_Openloop/Measurements/Speed, Acceleration, Direction and Angles Calculator/delta Thetae Calculator ==
  Speed (rpm) : Inport
  New Clock Time : Inport  Port=2
  Add : Sum  Inputs=+-
  Clock : Clock
      settings: Decimation=1000000
  Gain : Gain  Gain=(P*2*pi)/60
  Product : Product
  dThetae : Outport
  wires:
  New Clock Time/1 -> Add/2
  Clock/1 -> Add/1
  Gain/1 -> Product/2
  Product/1 -> dThetae/1
  Add/1 -> Product/1
  Speed (rpm)/1 -> Gain/1

== system BLDC_Openloop/Measurements/Torque & Flux calculator/dq_I_transform ==
  I_ab : Inport
  Demux : Demux  Outputs=2
  Gain : Gain  Gain=1/2  SaturateOnIntegerOverflow=on  OutDataTypeStr=Inherit: Same as input  ParamDataTypeStr=Inherit: Same as input
  Gain1 : Gain  Gain=1/2  SaturateOnIntegerOverflow=on  OutDataTypeStr=Inherit: Same as input  ParamDataTypeStr=Inherit: Same as input
  Gain2 : Gain  Gain=2/3  SaturateOnIntegerOverflow=on  OutDataTypeStr=Inherit: Same as input  ParamDataTypeStr=Inherit: Same as input
  Gain3 : Gain  Gain=sqrt(3)/2  SaturateOnIntegerOverflow=on  OutDataTypeStr=Inherit: Same as input  ParamDataTypeStr=Inherit: Same as input
  Gain4 : Gain  Gain=sqrt(3)/2  SaturateOnIntegerOverflow=on  OutDataTypeStr=Inherit: Same as input  ParamDataTypeStr=Inherit: Same as input
  Gain5 : Gain  Gain=2/3  SaturateOnIntegerOverflow=on  OutDataTypeStr=Inherit: Same as input  ParamDataTypeStr=Inherit: Same as input
  Sum2 : Sum  Inputs=-+  SaturateOnIntegerOverflow=on  InputSameDT=on  OutDataTypeStr=Inherit: Same as first input
  Sum3 : Sum  Inputs=+--  SaturateOnIntegerOverflow=on  InputSameDT=on  OutDataTypeStr=Inherit: Same as first input
  Sum4 : Sum  Inputs=--  SaturateOnIntegerOverflow=on  InputSameDT=on  OutDataTypeStr=Inherit: Same as first input
  I_q : Outport
  I_d : Outport  Port=2
  wires:
  Sum2/1 -> Gain5/1
  Gain4/1 -> Sum2/2
  Gain3/1 -> Sum2/1
  Sum3/1 -> Gain2/1
  Sum4/1 -> Gain4/1, Gain1/1
  Gain/1 -> Sum3/2
  Gain1/1 -> Sum3/3
  Demux/2 -> Sum4/2, Gain/1, Gain3/1
  Demux/1 -> Sum4/1, Sum3/1
  I_ab/1 -> Demux/1
  Gain5/1 -> I_d/1
  Gain2/1 -> I_q/1

== system BLDC_Openloop/Measurements/Torque & Flux calculator/dq_V_transform ==
  Vabc : Inport
  Demux : Demux  Outputs=3
  Gain : Gain  Gain=1/2  SaturateOnIntegerOverflow=on  OutDataTypeStr=Inherit: Same as input  ParamDataTypeStr=Inherit: Same as input
  Gain1 : Gain  Gain=1/2  SaturateOnIntegerOverflow=on  OutDataTypeStr=Inherit: Same as input  ParamDataTypeStr=Inherit: Same as input
  Gain2 : Gain  Gain=2/3  SaturateOnIntegerOverflow=on  OutDataTypeStr=Inherit: Same as input  ParamDataTypeStr=Inherit: Same as input
  Gain3 : Gain  Gain=sqrt(3)/2  SaturateOnIntegerOverflow=on  OutDataTypeStr=Inherit: Same as input  ParamDataTypeStr=Inherit: Same as input
  Gain4 : Gain  Gain=sqrt(3)/2  SaturateOnIntegerOverflow=on  OutDataTypeStr=Inherit: Same as input  ParamDataTypeStr=Inherit: Same as input
  Gain5 : Gain  Gain=2/3  SaturateOnIntegerOverflow=on  OutDataTypeStr=Inherit: Same as input  ParamDataTypeStr=Inherit: Same as input
  Sum2 : Sum  Inputs=+--  SaturateOnIntegerOverflow=on  InputSameDT=on  OutDataTypeStr=Inherit: Same as first input
  Sum3 : Sum  Inputs=-+  SaturateOnIntegerOverflow=on  InputSameDT=on  OutDataTypeStr=Inherit: Same as first input
  v_q : Outport
  v_d : Outport  Port=2
  wires:
  Sum3/1 -> Gain5/1
  Gain4/1 -> Sum3/2
  Gain3/1 -> Sum3/1
  Gain2/1 -> v_q/1
  Gain1/1 -> Sum2/3
  Gain/1 -> Sum2/2
  Demux/1 -> Sum2/1
  Sum2/1 -> Gain2/1
  Gain5/1 -> v_d/1
  Vabc/1 -> Demux/1
  Demux/2 -> Gain/1, Gain3/1
  Demux/3 -> Gain1/1, Gain4/1

== system BLDC_Openloop/Protection/MOSFET Failure Protection/Timer1 ==
  In1 : Inport
  Add2 : Sum  Inputs=+-
  C18 : simulink/Logic and Bit Operations/Compare To Constant  relop=>=  const=Risetimemax  OutDataTypeStr=boolean
  Clock : Clock
      settings: Decimation=1000000
  Compare To Zero : simulink/Logic and Bit Operations/Compare To Zero  relop===  OutDataTypeStr=boolean
  Switch : Switch  Threshold=1
  Out1 : Outport
  wires:
  Add2/1 -> C18/1
  In1/1 -> Compare To Zero/1
  Compare To Zero/1 -> Switch/2
  Switch/1 -> Switch/3, Add2/2
  Clock/1 -> Add2/1, Switch/1
  C18/1 -> Out1/1

== system BLDC_Openloop/Protection/MOSFET Failure Protection/Timer2 ==
  In1 : Inport
  Add2 : Sum  Inputs=+-
  C18 : simulink/Logic and Bit Operations/Compare To Constant  relop=>=  const=Risetimemax  OutDataTypeStr=boolean
  Clock : Clock
      settings: Decimation=1000000
  Compare To Zero : simulink/Logic and Bit Operations/Compare To Zero  relop===  OutDataTypeStr=boolean
  Switch : Switch  Threshold=1
  Out1 : Outport
  wires:
  Add2/1 -> C18/1
  In1/1 -> Compare To Zero/1
  Compare To Zero/1 -> Switch/2
  Switch/1 -> Switch/3, Add2/2
  Clock/1 -> Add2/1, Switch/1
  C18/1 -> Out1/1

== system BLDC_Openloop/Protection/MOSFET Failure Protection/Timer4 ==
  In1 : Inport
  Add2 : Sum  Inputs=+-
  C18 : simulink/Logic and Bit Operations/Compare To Constant  relop=>=  const=Risetimemax  OutDataTypeStr=boolean
  Clock : Clock
      settings: Decimation=1000000
  Compare To Zero : simulink/Logic and Bit Operations/Compare To Zero  relop===  OutDataTypeStr=boolean
  Switch : Switch  Threshold=1
  Out1 : Outport
  wires:
  Add2/1 -> C18/1
  In1/1 -> Compare To Zero/1
  Compare To Zero/1 -> Switch/2
  Switch/1 -> Switch/3, Add2/2
  Clock/1 -> Add2/1, Switch/1
  C18/1 -> Out1/1
